simulink model "Research_project_CSTR_cascade"  (R2022b)
settings: Solver=ode23s  StartTime=0.0  StopTime=360  RelTol=1e-3
model workspace (MAT data in the model file):
  Var = 0
undefined symbols (not defined in the file): A, CA0, FA0, Tfeed, Tfeedout, Tj, U, V, v0, Xin, Xout
(part 2 of 2)

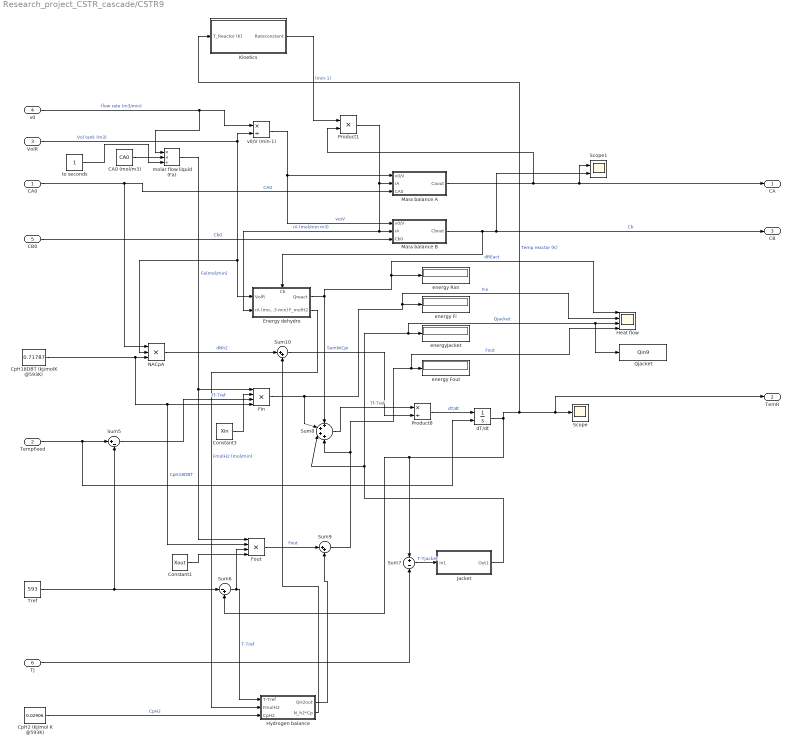
== system Research_project_CSTR_cascade/CSTR9 ==
  CA0 : Inport
  TempFeed : Inport  Port=2
  VolR : Inport  Port=3
  v0 : Inport  Port=4
  CB0 : Inport  Port=5
  Tj : Inport  Port=6
  CA0 (mol/m3) : Constant  Value=CA0
  Constant1 : Constant  Value=Xout
  Constant3 : Constant  Value=Xin
  CpH18DBT (kj/molK @593K) : Constant  Value=0.71787
  CpH2 (kj/mol K @593K) : Constant  Value=0.02906
  Energy dehydro : Subsystem
      settings: PortSchema="{\"entries\":[{\"content\":{\"sides\":[{\"content\":{\"connectorIds\":[\"In1\",\"In2\"]},\"type\":\"ConnectorPlacement.EquallySpacedRectSide\",\"uuid\":\"ea2ca829-97b9-403b-8ba1-0454ae3e30fe\"},{\"content\":{\"connectorIds\":[\"Out1\",\"Out2\"],\"side\":\"RIGHT\"},\"type\":\"ConnectorPlacement.EquallySpacedRectSide\",\"uuid\":\"58c9b242-3f0e-4d7f-8153-41ceacc042f7\"},{\"content\":{\"connectorIds\":[\"In3\"],\"side\":\"TOP\"},\"type\":\"ConnectorPlacement.EquallySpacedRectSide\",\"uuid\":\"130a98c9-d360-4861-8a60-9ab6de0c7020\"}]},\"type\":\"ConnectorPlacement.EquallySpacedConnector\",\"uuid\":\"a36fbf0c-f6b7-4cf9-83b8-7faebe270894\"}],\"packageUris\":[\"http://schema.mathworks.com/mf0/Connector/R2020b\"],\"version\":\"1.0\"}"
  Fin : Product  Inputs=4
  Fout : Product  Inputs=4
  Heat flow : Scope  NumInputPorts=4
  Hydrogen balance : Subsystem
  Jacket : Subsystem
  Kinetics : Subsystem
  Mass balance A : Subsystem
  Mass balance B : Subsystem
  NACpA : Product  Inputs=3
  Product1 : Product
  Product8 : Product  Inputs=*/
  Qjacket : ToWorkspace  VariableName=Qin9  SaveFormat=Timeseries  SampleTime=1
  Scope : Scope
  Scope1 : Scope  NumInputPorts=2
  Sum10 : Sum  Inputs=|++
  Sum5 : Sum  Inputs=|+-
  Sum6 : Sum  Inputs=|-+
  Sum7 : Sum  Inputs=+-
  Sum8 : Sum  Inputs=++++
  Sum9 : Sum  Inputs=|++
  Tref : Constant  Value=593
  dT/dt : Integrator  InitialConditionSource=external  InitialCondition=593
  energy Fi : Display
  energy Fout : Display
  energy Rxn : Display
  energyJacket : Display
  molar flow liquid (Fa) : Product  Inputs=**/
  to seconds : Constant
  v0/V (min-1) : Product  Inputs=*/
  CA : Outport
  TemR : Outport  Port=2
  CB : Outport  Port=3
  wires:
  VolR/1 -> Energy dehydro/1(VolR), NACpA/2, v0/V (min-1)/2  "Vol tank (m3)"
  v0/1 -> v0/V (min-1)/1, molar flow liquid (Fa)/1  "flow rate (m3/min)"
  CA0/1 -> NACpA/1, Mass balance A/3(CA0)  "CA0"
  Product1/1 -> Mass balance A/2(rA), Energy dehydro/2(rA (mol/m3 min)), Mass balance B/2(rA)  "rA (mol/min m3)"
  CB0/1 -> Mass balance B/3(Cb0)  "Cb0"
  v0/V (min-1)/1 -> Mass balance B/1(v0/V), Mass balance A/1(v0/V)  "vo/V"
  Mass balance B/1(Cbout) -> CB/1, Scope1/2, Energy dehydro/3(Cb)  "Cb"
  CpH18DBT (kj/molK @593K)/1 -> NACpA/3, Fin/4, Fout/2  "CpH18DBT"
  Tref/1 -> Sum5/2, Sum6/1
  Sum5/1 -> Fin/3  "Tf-Tref"
  to seconds/1 -> molar flow liquid (Fa)/3
  molar flow liquid (Fa)/1 -> Fout/1, Fin/1  "Fa(mol/min)"
  dT/dt/1 -> Kinetics/1(T_Reactor (K)), TemR/1, Scope/1, Sum6/2, Sum7/1  "Temp reactor (K)"
  Sum6/1 -> Hydrogen balance/1(T-Tref), Fout/3  "T-Tref"
  Tj/1 -> Sum7/2
  Jacket/1(Out1) -> Qjacket/1, Heat flow/3, energyJacket/1, Sum8/3  "Qjacket"
  Fin/1 -> Heat flow/2, energy Fi/1, Sum8/2  "Fin"
  Sum9/1 -> Heat flow/4, energy Fout/1, Sum8/4  "Fout"
  Energy dehydro/1(Qreact) -> Sum8/1, Heat flow/1, energy Rxn/1  "dREact"
  Sum8/1 -> Product8/1  "Tf-Tref"
  Product8/1 -> dT/dt/1  "dT/dt"
  Constant1/1 -> Fout/4
  TempFeed/1 -> dT/dt/2, Sum5/1
  Kinetics/1(Rateconstant) -> Product1/1  "(min-1)"
  Constant3/1 -> Fin/2
  CpH2 (kj/mol K @593K)/1 -> Hydrogen balance/3(CpH2)  "CpH2"
  Energy dehydro/2(F_molH2) -> Hydrogen balance/2(FmolH2)  "FmolH2 (mol/min)"
  Fout/1 -> Sum9/1  "Fout"
  Sum7/1 -> Jacket/1(In1)  "T-Tjacket"
  Hydrogen balance/1(QH2out) -> Sum9/2
  NACpA/1 -> Sum10/1  "dNh2"
  Sum10/1 -> Product8/2  "SumNiCpi"
  Hydrogen balance/2(N_h2*Cp) -> Sum10/2
  Mass balance A/1(Caout) -> Scope1/1, CA/1, Product1/2
  CA0 (mol/m3)/1 -> molar flow liquid (Fa)/2

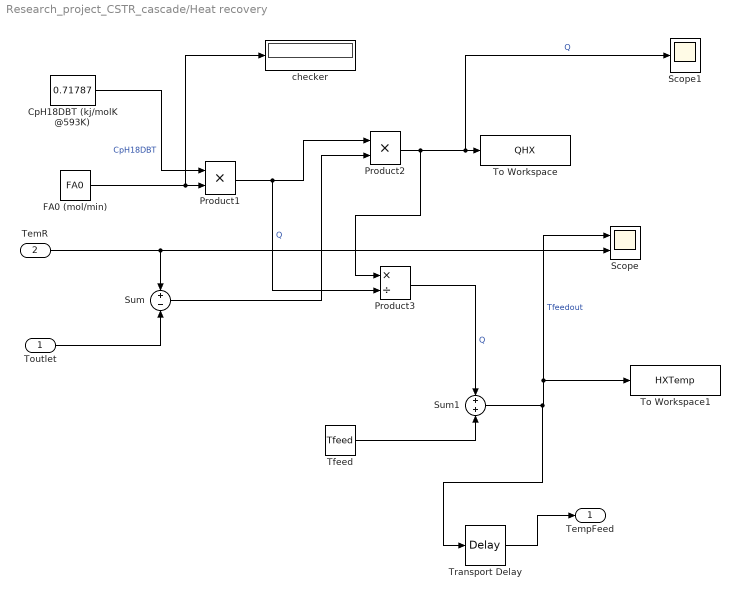
== system Research_project_CSTR_cascade/Heat recovery ==
  Toutlet : Inport
  TemR : Inport  Port=2
  CpH18DBT (kj/molK @593K) : Constant  Value=0.71787
  FA0 (mol/min) : Constant  Value=FA0
  Product1 : Product
  Product2 : Product
  Product3 : Product  Inputs=*/
  Scope : Scope  NumInputPorts=2
  Scope1 : Scope
  Sum : Sum  Inputs=+-
  Sum1 : Sum
  Tfeed : Constant  Value=Tfeed
  To Workspace : ToWorkspace  VariableName=QHX  SaveFormat=Timeseries  SampleTime=1
  To Workspace1 : ToWorkspace  VariableName=HXTemp  SaveFormat=Timeseries  SampleTime=5
  Transport Delay : TransportDelay
  checker : Display
  TempFeed : Outport
  wires:
  TemR/1 -> Sum/1, Scope/2
  FA0 (mol/min)/1 -> checker/1, Product1/2
  Sum/1 -> Product2/2
  CpH18DBT (kj/molK @593K)/1 -> Product1/1  "CpH18DBT"
  Product2/1 -> Product3/1, Scope1/1, To Workspace/1  "Q"
  Product1/1 -> Product3/2, Product2/1  "Q"
  Tfeed/1 -> Sum1/2
  Product3/1 -> Sum1/1  "Q"
  Sum1/1 -> Transport Delay/1, To Workspace1/1, Scope/1  "Tfeedout"
  Transport Delay/1 -> TempFeed/1
  Toutlet/1 -> Sum/2

== system Research_project_CSTR_cascade/mol ==
  V : Inport
  Cb : Inport  Port=2
  CA : Inport  Port=3
  Constant : Constant  Value=9
  Product : Product
  Product1 : Product
  Product2 : Product
  H2 : Outport
  H0DBT : Outport  Port=2
  H18DBT : Outport  Port=3
  wires:
  Product1/1 -> H0DBT/1, Product2/2  "H0DBT"
  Constant/1 -> Product2/1
  Product/1 -> H18DBT/1  "H18DBT"
  Product2/1 -> H2/1  "H2"
  V/1 -> Product1/1, Product/1  "V"
  CA/1 -> Product/2  "Conc H18-DBT"
  Cb/1 -> Product1/2

== system Research_project_CSTR_cascade/CSTR1/Energy dehydro ==
  VolR : Inport
  rA (mol/m3 min) : Inport  Port=2
  Cb : Inport  Port=3
  9H2 : Constant  Value=9
  Product1 : Product  Inputs=3
  Product2 : Product  Inputs=3
  Product6 : Product
  reaction enth (kj/molH2) : Constant  Value=-64
  Qreact : Outport
  F_molH2 : Outport  Port=2
  wires:
  9H2/1 -> Product2/2, Product1/3
  VolR/1 -> Product2/1, Product1/1
  rA (mol/m3 min)/1 -> Product1/2
  reaction enth (kj/molH2)/1 -> Product6/2
  Product1/1 -> F_molH2/1, Product6/1  "rA rate of H2 react (mol of H2/min)"
  Product6/1 -> Qreact/1  "dREact"
  Cb/1 -> Product2/3  "mol/m3min"

== system Research_project_CSTR_cascade/CSTR1/Hydrogen balance ==
  T-Tref : Inport
  FmolH2 : Inport  Port=2
  CpH2 : Inport  Port=3
  Constant1 : Constant  Value=Xout
  FoutH2CpdT2 : Product  Inputs=4
  N_H2*Cp : Product
  Scope1 : Scope
  QH2out : Outport
  N_h2*Cp : Outport  Port=2
  wires:
  FoutH2CpdT2/1 -> Scope1/1, QH2out/1  "QH2"
  T-Tref/1 -> FoutH2CpdT2/1
  CpH2/1 -> N_H2*Cp/2, FoutH2CpdT2/2
  FmolH2/1 -> N_H2*Cp/1, FoutH2CpdT2/3
  N_H2*Cp/1 -> N_h2*Cp/1  "QH2"
  Constant1/1 -> FoutH2CpdT2/4

== system Research_project_CSTR_cascade/CSTR1/Jacket ==
  In1 : Inport
  Area Heat (m2) : Constant  Value=A
  Q : Product  Inputs=3
  U (Kj/min m2 K) : Constant  Value=U
  Out1 : Outport
  wires:
  Area Heat (m2)/1 -> Q/3  "A jacket (m2)"
  U (Kj/min m2 K)/1 -> Q/1
  In1/1 -> Q/2  "T-Tjacket"
  Q/1 -> Out1/1  "Qjacket"

== system Research_project_CSTR_cascade/CSTR1/Kinetics ==
  T_Reactor (K) : Inport
  "A constant " : Math
  Constant : Constant  Value=37.634
  Ea (kj/mol) : Constant  Value=-204.68
  Effectiveness factor : Constant
  Math Function : Math
  Product3 : Product
  Product4 : Product  Inputs=3
  Product5 : Product  Inputs=*/
  R (kj/mol K) : Constant  Value=0.00831
  Rateconstant : Outport
  wires:
  T_Reactor (K)/1 -> Product3/1
  "A constant "/1 -> Product4/1
  Product3/1 -> Product5/2
  Constant/1 -> "A constant "/1
  Ea (kj/mol)/1 -> Product5/1
  Math Function/1 -> Product4/2
  R (kj/mol K)/1 -> Product3/2
  Product5/1 -> Math Function/1
  Product4/1 -> Rateconstant/1  "(min-1)"
  Effectiveness factor/1 -> Product4/3

== system Research_project_CSTR_cascade/CSTR1/Mass balance A ==
  v0/V : Inport
  rA : Inport  Port=2
  CA0 : Inport  Port=3
  Product1 : Product
  Scope : Scope
  Sum1 : Sum  Inputs=|+-
  Sum2 : Sum  Inputs=|+-
  dCa/dt : Integrator  InitialConditionSource=external  InitialCondition=3100
  Caout : Outport
  wires:
  rA/1 -> Sum2/2  "rA (mol/min m3)"
  Sum2/1 -> dCa/dt/1
  CA0/1 -> dCa/dt/2, Sum1/1
  Product1/1 -> Sum2/1
  dCa/dt/1 -> Scope/1, Caout/1, Sum1/2  "Ca (mol/m3 min)"
  Sum1/1 -> Product1/2  "Ca0-Ca"
  v0/V/1 -> Product1/1

== system Research_project_CSTR_cascade/CSTR1/Mass balance B ==
  v0/V : Inport
  rA : Inport  Port=2
  Cb0 : Inport  Port=3
  Product1 : Product
  Scope : Scope
  Sum1 : Sum  Inputs=|+-
  Sum2 : Sum  Inputs=|++
  dCb/dt : Integrator  InitialConditionSource=external  InitialCondition=3100
  Cbout : Outport
  wires:
  rA/1 -> Sum2/2  "rA (mol/min m3)"
  Sum2/1 -> dCb/dt/1
  Cb0/1 -> dCb/dt/2, Sum1/1
  Product1/1 -> Sum2/1
  dCb/dt/1 -> Scope/1, Cbout/1, Sum1/2  "Cb (mol/m3 min)"
  Sum1/1 -> Product1/2  "Cb0-Cb"
  v0/V/1 -> Product1/1

== system Research_project_CSTR_cascade/CSTR10/Energy dehydro ==
  VolR : Inport
  rA (mol/m3 min) : Inport  Port=2
  9H2 : Constant  Value=9
  B : Constant
  Product1 : Product  Inputs=3
  Product2 : Product  Inputs=3
  Product6 : Product
  Qjacket : ToWorkspace  VariableName=H2  SaveFormat=Timeseries  SampleTime=5
  Scope1 : Scope  NumInputPorts=2
  reaction enth (kj/molH2) : Constant  Value=-64
  Qreact : Outport
  F_molH2 : Outport  Port=2
  wires:
  9H2/1 -> Product1/3
  VolR/1 -> Product2/1, Product1/1
  rA (mol/m3 min)/1 -> Product2/2, Product1/2
  reaction enth (kj/molH2)/1 -> Product6/2
  Product6/1 -> Qreact/1  "dREact"
  Product1/1 -> Qjacket/1, Scope1/2, F_molH2/1, Product6/1  "mol of H2"
  Product2/1 -> Scope1/1  "mol H0-DBT"
  B/1 -> Product2/3

== system Research_project_CSTR_cascade/CSTR10/Hydrogen balance ==
  T-Tref : Inport
  FmolH2 : Inport  Port=2
  CpH2 : Inport  Port=3
  Constant1 : Constant  Value=Xout
  FoutH2CpdT2 : Product  Inputs=4
  N_H2*Cp : Product
  Scope1 : Scope
  QH2out : Outport
  N_h2*Cp : Outport  Port=2
  wires:
  FoutH2CpdT2/1 -> Scope1/1, QH2out/1  "QH2"
  T-Tref/1 -> FoutH2CpdT2/1
  CpH2/1 -> N_H2*Cp/2, FoutH2CpdT2/2
  FmolH2/1 -> N_H2*Cp/1, FoutH2CpdT2/3
  N_H2*Cp/1 -> N_h2*Cp/1  "QH2"
  Constant1/1 -> FoutH2CpdT2/4

== system Research_project_CSTR_cascade/CSTR10/Jacket ==
  In1 : Inport
  Area Heat (m2) : Constant  Value=A
  Q : Product  Inputs=3
  U (Kj/min m2 K) : Constant  Value=U
  Out1 : Outport
  wires:
  Area Heat (m2)/1 -> Q/3  "A jacket (m2)"
  U (Kj/min m2 K)/1 -> Q/1
  In1/1 -> Q/2  "T-Tjacket"
  Q/1 -> Out1/1  "Qjacket"

== system Research_project_CSTR_cascade/CSTR10/Kinetics ==
  T_Reactor (K) : Inport
  "A constant " : Math
  Constant : Constant  Value=37.634
  Ea (kj/mol) : Constant  Value=-204.68
  Effectiveness factor : Constant
  Math Function : Math
  Product3 : Product
  Product4 : Product  Inputs=3
  Product5 : Product  Inputs=*/
  R (kj/mol K) : Constant  Value=0.00831
  Rateconstant : Outport
  wires:
  T_Reactor (K)/1 -> Product3/1
  "A constant "/1 -> Product4/1
  Product3/1 -> Product5/2
  Constant/1 -> "A constant "/1
  Ea (kj/mol)/1 -> Product5/1
  Math Function/1 -> Product4/2
  R (kj/mol K)/1 -> Product3/2
  Product5/1 -> Math Function/1
  Product4/1 -> Rateconstant/1  "(min-1)"
  Effectiveness factor/1 -> Product4/3

== system Research_project_CSTR_cascade/CSTR10/Mass balance A ==
  v0/V : Inport
  rA : Inport  Port=2
  CA0 : Inport  Port=3
  Product1 : Product
  Scope : Scope
  Sum1 : Sum  Inputs=|+-
  Sum2 : Sum  Inputs=|+-
  dCa/dt : Integrator  InitialConditionSource=external  InitialCondition=3100
  Caout : Outport
  wires:
  rA/1 -> Sum2/2  "rA (mol/min m3)"
  Sum2/1 -> dCa/dt/1
  CA0/1 -> dCa/dt/2, Sum1/1
  Product1/1 -> Sum2/1
  dCa/dt/1 -> Scope/1, Caout/1, Sum1/2  "Ca (mol/m3 min)"
  Sum1/1 -> Product1/2  "Ca0-Ca"
  v0/V/1 -> Product1/1

== system Research_project_CSTR_cascade/CSTR10/Mass balance B ==
  v0/V : Inport
  rA : Inport  Port=2
  Cb0 : Inport  Port=3
  Product1 : Product
  Scope : Scope
  Sum1 : Sum  Inputs=|+-
  Sum2 : Sum  Inputs=|++
  dCb/dt : Integrator  InitialConditionSource=external  InitialCondition=3100
  Cbout : Outport
  wires:
  rA/1 -> Sum2/2  "rA (mol/min m3)"
  Sum2/1 -> dCb/dt/1
  Cb0/1 -> dCb/dt/2, Sum1/1
  Product1/1 -> Sum2/1
  dCb/dt/1 -> Scope/1, Cbout/1, Sum1/2  "Cb (mol/m3 min)"
  Sum1/1 -> Product1/2  "Cb0-Cb"
  v0/V/1 -> Product1/1

== system Research_project_CSTR_cascade/CSTR2/Energy dehydro ==
  VolR : Inport
  rA (mol/m3 min) : Inport  Port=2
  Cb : Inport  Port=3
  9H2 : Constant  Value=9
  Product1 : Product  Inputs=3
  Product2 : Product  Inputs=3
  Product6 : Product
  reaction enth (kj/molH2) : Constant  Value=-64
  Qreact : Outport
  F_molH2 : Outport  Port=2
  wires:
  9H2/1 -> Product2/2, Product1/3
  VolR/1 -> Product2/1, Product1/1
  rA (mol/m3 min)/1 -> Product1/2
  reaction enth (kj/molH2)/1 -> Product6/2
  Product1/1 -> F_molH2/1, Product6/1  "rA rate of H2 react (mol of H2/min)"
  Product6/1 -> Qreact/1  "dREact"
  Cb/1 -> Product2/3  "mol/m3min"

== system Research_project_CSTR_cascade/CSTR2/Hydrogen balance ==
  T-Tref : Inport
  FmolH2 : Inport  Port=2
  CpH2 : Inport  Port=3
  Constant1 : Constant  Value=Xout
  FoutH2CpdT2 : Product  Inputs=4
  N_H2*Cp : Product
  Scope1 : Scope
  QH2out : Outport
  N_h2*Cp : Outport  Port=2
  wires:
  FoutH2CpdT2/1 -> Scope1/1, QH2out/1  "QH2"
  T-Tref/1 -> FoutH2CpdT2/1
  CpH2/1 -> N_H2*Cp/2, FoutH2CpdT2/2
  FmolH2/1 -> N_H2*Cp/1, FoutH2CpdT2/3
  N_H2*Cp/1 -> N_h2*Cp/1  "QH2"
  Constant1/1 -> FoutH2CpdT2/4

== system Research_project_CSTR_cascade/CSTR2/Jacket ==
  In1 : Inport
  Area Heat (m2) : Constant  Value=A
  Q : Product  Inputs=3
  U (Kj/min m2 K) : Constant  Value=U
  Out1 : Outport
  wires:
  Area Heat (m2)/1 -> Q/3  "A jacket (m2)"
  U (Kj/min m2 K)/1 -> Q/1
  In1/1 -> Q/2  "T-Tjacket"
  Q/1 -> Out1/1  "Qjacket"

== system Research_project_CSTR_cascade/CSTR2/Kinetics ==
  T_Reactor (K) : Inport
  "A constant " : Math
  Constant : Constant  Value=37.634
  Ea (kj/mol) : Constant  Value=-204.68
  Effectiveness factor : Constant
  Math Function : Math
  Product3 : Product
  Product4 : Product  Inputs=3
  Product5 : Product  Inputs=*/
  R (kj/mol K) : Constant  Value=0.00831
  Rateconstant : Outport
  wires:
  T_Reactor (K)/1 -> Product3/1
  "A constant "/1 -> Product4/1
  Product3/1 -> Product5/2
  Constant/1 -> "A constant "/1
  Ea (kj/mol)/1 -> Product5/1
  Math Function/1 -> Product4/2
  R (kj/mol K)/1 -> Product3/2
  Product5/1 -> Math Function/1
  Product4/1 -> Rateconstant/1  "(min-1)"
  Effectiveness factor/1 -> Product4/3

== system Research_project_CSTR_cascade/CSTR2/Mass balance A ==
  v0/V : Inport
  rA : Inport  Port=2
  CA0 : Inport  Port=3
  Product1 : Product
  Scope : Scope
  Sum1 : Sum  Inputs=|+-
  Sum2 : Sum  Inputs=|+-
  dCa/dt : Integrator  InitialConditionSource=external  InitialCondition=3100
  Caout : Outport
  wires:
  rA/1 -> Sum2/2  "rA (mol/min m3)"
  Sum2/1 -> dCa/dt/1
  CA0/1 -> dCa/dt/2, Sum1/1
  Product1/1 -> Sum2/1
  dCa/dt/1 -> Scope/1, Caout/1, Sum1/2  "Ca (mol/m3 min)"
  Sum1/1 -> Product1/2  "Ca0-Ca"
  v0/V/1 -> Product1/1

== system Research_project_CSTR_cascade/CSTR2/Mass balance B ==
  v0/V : Inport
  rA : Inport  Port=2
  Cb0 : Inport  Port=3
  Product1 : Product
  Scope : Scope
  Sum1 : Sum  Inputs=|+-
  Sum2 : Sum  Inputs=|++
  dCb/dt : Integrator  InitialConditionSource=external  InitialCondition=3100
  Cbout : Outport
  wires:
  rA/1 -> Sum2/2  "rA (mol/min m3)"
  Sum2/1 -> dCb/dt/1
  Cb0/1 -> dCb/dt/2, Sum1/1
  Product1/1 -> Sum2/1
  dCb/dt/1 -> Scope/1, Cbout/1, Sum1/2  "Cb (mol/m3 min)"
  Sum1/1 -> Product1/2  "Cb0-Cb"
  v0/V/1 -> Product1/1

== system Research_project_CSTR_cascade/CSTR3/Energy dehydro ==
  VolR : Inport
  rA (mol/m3 min) : Inport  Port=2
  Cb : Inport  Port=3
  9H2 : Constant  Value=9
  Product1 : Product  Inputs=3
  Product2 : Product  Inputs=3
  Product6 : Product
  reaction enth (kj/molH2) : Constant  Value=-64
  Qreact : Outport
  F_molH2 : Outport  Port=2
  wires:
  9H2/1 -> Product2/2, Product1/3
  VolR/1 -> Product2/1, Product1/1
  rA (mol/m3 min)/1 -> Product1/2
  reaction enth (kj/molH2)/1 -> Product6/2
  Product1/1 -> F_molH2/1, Product6/1  "rA rate of H2 react (mol of H2/min)"
  Product6/1 -> Qreact/1  "dREact"
  Cb/1 -> Product2/3  "mol/m3min"

== system Research_project_CSTR_cascade/CSTR3/Hydrogen balance ==
  T-Tref : Inport
  FmolH2 : Inport  Port=2
  CpH2 : Inport  Port=3
  Constant1 : Constant  Value=Xout
  FoutH2CpdT2 : Product  Inputs=4
  N_H2*Cp : Product
  Scope1 : Scope
  QH2out : Outport
  N_h2*Cp : Outport  Port=2
  wires:
  FoutH2CpdT2/1 -> Scope1/1, QH2out/1  "QH2"
  T-Tref/1 -> FoutH2CpdT2/1
  CpH2/1 -> N_H2*Cp/2, FoutH2CpdT2/2
  FmolH2/1 -> N_H2*Cp/1, FoutH2CpdT2/3
  N_H2*Cp/1 -> N_h2*Cp/1  "QH2"
  Constant1/1 -> FoutH2CpdT2/4

== system Research_project_CSTR_cascade/CSTR3/Jacket ==
  In1 : Inport
  Area Heat (m2) : Constant  Value=A
  Q : Product  Inputs=3
  U (Kj/min m2 K) : Constant  Value=U
  Out1 : Outport
  wires:
  Area Heat (m2)/1 -> Q/3  "A jacket (m2)"
  U (Kj/min m2 K)/1 -> Q/1
  In1/1 -> Q/2  "T-Tjacket"
  Q/1 -> Out1/1  "Qjacket"

== system Research_project_CSTR_cascade/CSTR3/Kinetics ==
  T_Reactor (K) : Inport
  "A constant " : Math
  Constant : Constant  Value=37.634
  Ea (kj/mol) : Constant  Value=-204.68
  Effectiveness factor : Constant
  Math Function : Math
  Product3 : Product
  Product4 : Product  Inputs=3
  Product5 : Product  Inputs=*/
  R (kj/mol K) : Constant  Value=0.00831
  Rateconstant : Outport
  wires:
  T_Reactor (K)/1 -> Product3/1
  "A constant "/1 -> Product4/1
  Product3/1 -> Product5/2
  Constant/1 -> "A constant "/1
  Ea (kj/mol)/1 -> Product5/1
  Math Function/1 -> Product4/2
  R (kj/mol K)/1 -> Product3/2
  Product5/1 -> Math Function/1
  Product4/1 -> Rateconstant/1  "(min-1)"
  Effectiveness factor/1 -> Product4/3

== system Research_project_CSTR_cascade/CSTR3/Mass balance A ==
  v0/V : Inport
  rA : Inport  Port=2
  CA0 : Inport  Port=3
  Product1 : Product
  Scope : Scope
  Sum1 : Sum  Inputs=|+-
  Sum2 : Sum  Inputs=|+-
  dCa/dt : Integrator  InitialConditionSource=external  InitialCondition=3100
  Caout : Outport
  wires:
  rA/1 -> Sum2/2  "rA (mol/min m3)"
  Sum2/1 -> dCa/dt/1
  CA0/1 -> dCa/dt/2, Sum1/1
  Product1/1 -> Sum2/1
  dCa/dt/1 -> Scope/1, Caout/1, Sum1/2  "Ca (mol/m3 min)"
  Sum1/1 -> Product1/2  "Ca0-Ca"
  v0/V/1 -> Product1/1

== system Research_project_CSTR_cascade/CSTR3/Mass balance B ==
  v0/V : Inport
  rA : Inport  Port=2
  Cb0 : Inport  Port=3
  Product1 : Product
  Scope : Scope
  Sum1 : Sum  Inputs=|+-
  Sum2 : Sum  Inputs=|++
  dCb/dt : Integrator  InitialConditionSource=external  InitialCondition=3100
  Cbout : Outport
  wires:
  rA/1 -> Sum2/2  "rA (mol/min m3)"
  Sum2/1 -> dCb/dt/1
  Cb0/1 -> dCb/dt/2, Sum1/1
  Product1/1 -> Sum2/1
  dCb/dt/1 -> Scope/1, Cbout/1, Sum1/2  "Cb (mol/m3 min)"
  Sum1/1 -> Product1/2  "Cb0-Cb"
  v0/V/1 -> Product1/1

== system Research_project_CSTR_cascade/CSTR4/Energy dehydro ==
  VolR : Inport
  rA (mol/m3 min) : Inport  Port=2
  Cb : Inport  Port=3
  9H2 : Constant  Value=9
  Product1 : Product  Inputs=3
  Product2 : Product  Inputs=3
  Product6 : Product
  reaction enth (kj/molH2) : Constant  Value=-64
  Qreact : Outport
  F_molH2 : Outport  Port=2
  wires:
  9H2/1 -> Product2/2, Product1/3
  VolR/1 -> Product2/1, Product1/1
  rA (mol/m3 min)/1 -> Product1/2
  reaction enth (kj/molH2)/1 -> Product6/2
  Product1/1 -> F_molH2/1, Product6/1  "rA rate of H2 react (mol of H2/min)"
  Product6/1 -> Qreact/1  "dREact"
  Cb/1 -> Product2/3  "mol/m3min"

== system Research_project_CSTR_cascade/CSTR4/Hydrogen balance ==
  T-Tref : Inport
  FmolH2 : Inport  Port=2
  CpH2 : Inport  Port=3
  Constant1 : Constant  Value=Xout
  FoutH2CpdT2 : Product  Inputs=4
  N_H2*Cp : Product
  Scope1 : Scope
  QH2out : Outport
  N_h2*Cp : Outport  Port=2
  wires:
  FoutH2CpdT2/1 -> Scope1/1, QH2out/1  "QH2"
  T-Tref/1 -> FoutH2CpdT2/1
  CpH2/1 -> N_H2*Cp/2, FoutH2CpdT2/2
  FmolH2/1 -> N_H2*Cp/1, FoutH2CpdT2/3
  N_H2*Cp/1 -> N_h2*Cp/1  "QH2"
  Constant1/1 -> FoutH2CpdT2/4

== system Research_project_CSTR_cascade/CSTR4/Jacket ==
  In1 : Inport
  Area Heat (m2) : Constant  Value=A
  Q : Product  Inputs=3
  U (Kj/min m2 K) : Constant  Value=U
  Out1 : Outport
  wires:
  Area Heat (m2)/1 -> Q/3  "A jacket (m2)"
  U (Kj/min m2 K)/1 -> Q/1
  In1/1 -> Q/2  "T-Tjacket"
  Q/1 -> Out1/1  "Qjacket"

== system Research_project_CSTR_cascade/CSTR4/Kinetics ==
  T_Reactor (K) : Inport
  "A constant " : Math
  Constant : Constant  Value=37.634
  Ea (kj/mol) : Constant  Value=-204.68
  Effectiveness factor : Constant
  Math Function : Math
  Product3 : Product
  Product4 : Product  Inputs=3
  Product5 : Product  Inputs=*/
  R (kj/mol K) : Constant  Value=0.00831
  Rateconstant : Outport
  wires:
  T_Reactor (K)/1 -> Product3/1
  "A constant "/1 -> Product4/1
  Product3/1 -> Product5/2
  Constant/1 -> "A constant "/1
  Ea (kj/mol)/1 -> Product5/1
  Math Function/1 -> Product4/2
  R (kj/mol K)/1 -> Product3/2
  Product5/1 -> Math Function/1
  Product4/1 -> Rateconstant/1  "(min-1)"
  Effectiveness factor/1 -> Product4/3

== system Research_project_CSTR_cascade/CSTR4/Mass balance A ==
  v0/V : Inport
  rA : Inport  Port=2
  CA0 : Inport  Port=3
  Product1 : Product
  Scope : Scope
  Sum1 : Sum  Inputs=|+-
  Sum2 : Sum  Inputs=|+-
  dCa/dt : Integrator  InitialConditionSource=external  InitialCondition=3100
  Caout : Outport
  wires:
  rA/1 -> Sum2/2  "rA (mol/min m3)"
  Sum2/1 -> dCa/dt/1
  CA0/1 -> dCa/dt/2, Sum1/1
  Product1/1 -> Sum2/1
  dCa/dt/1 -> Scope/1, Caout/1, Sum1/2  "Ca (mol/m3 min)"
  Sum1/1 -> Product1/2  "Ca0-Ca"
  v0/V/1 -> Product1/1

== system Research_project_CSTR_cascade/CSTR4/Mass balance B ==
  v0/V : Inport
  rA : Inport  Port=2
  Cb0 : Inport  Port=3
  Product1 : Product
  Scope : Scope
  Sum1 : Sum  Inputs=|+-
  Sum2 : Sum  Inputs=|++
  dCb/dt : Integrator  InitialConditionSource=external  InitialCondition=3100
  Cbout : Outport
  wires:
  rA/1 -> Sum2/2  "rA (mol/min m3)"
  Sum2/1 -> dCb/dt/1
  Cb0/1 -> dCb/dt/2, Sum1/1
  Product1/1 -> Sum2/1
  dCb/dt/1 -> Scope/1, Cbout/1, Sum1/2  "Cb (mol/m3 min)"
  Sum1/1 -> Product1/2  "Cb0-Cb"
  v0/V/1 -> Product1/1

== system Research_project_CSTR_cascade/CSTR5/Energy dehydro ==
  VolR : Inport
  rA (mol/m3 min) : Inport  Port=2
  Cb : Inport  Port=3
  9H2 : Constant  Value=9
  Product1 : Product  Inputs=3
  Product2 : Product  Inputs=3
  Product6 : Product
  reaction enth (kj/molH2) : Constant  Value=-64
  Qreact : Outport
  F_molH2 : Outport  Port=2
  wires:
  9H2/1 -> Product2/2, Product1/3
  VolR/1 -> Product2/1, Product1/1
  rA (mol/m3 min)/1 -> Product1/2
  reaction enth (kj/molH2)/1 -> Product6/2
  Product1/1 -> F_molH2/1, Product6/1  "rA rate of H2 react (mol of H2/min)"
  Product6/1 -> Qreact/1  "dREact"
  Cb/1 -> Product2/3  "mol/m3min"

== system Research_project_CSTR_cascade/CSTR5/Hydrogen balance ==
  T-Tref : Inport
  FmolH2 : Inport  Port=2
  CpH2 : Inport  Port=3
  Constant1 : Constant  Value=Xout
  FoutH2CpdT2 : Product  Inputs=4
  N_H2*Cp : Product
  Scope1 : Scope
  QH2out : Outport
  N_h2*Cp : Outport  Port=2
  wires:
  FoutH2CpdT2/1 -> Scope1/1, QH2out/1  "QH2"
  T-Tref/1 -> FoutH2CpdT2/1
  CpH2/1 -> N_H2*Cp/2, FoutH2CpdT2/2
  FmolH2/1 -> N_H2*Cp/1, FoutH2CpdT2/3
  N_H2*Cp/1 -> N_h2*Cp/1  "QH2"
  Constant1/1 -> FoutH2CpdT2/4

== system Research_project_CSTR_cascade/CSTR5/Jacket ==
  In1 : Inport
  Area Heat (m2) : Constant  Value=A
  Q : Product  Inputs=3
  U (Kj/min m2 K) : Constant  Value=U
  Out1 : Outport
  wires:
  Area Heat (m2)/1 -> Q/3  "A jacket (m2)"
  U (Kj/min m2 K)/1 -> Q/1
  In1/1 -> Q/2  "T-Tjacket"
  Q/1 -> Out1/1  "Qjacket"

== system Research_project_CSTR_cascade/CSTR5/Kinetics ==
  T_Reactor (K) : Inport
  "A constant " : Math
  Constant : Constant  Value=37.634
  Ea (kj/mol) : Constant  Value=-204.68
  Effectiveness factor : Constant
  Math Function : Math
  Product3 : Product
  Product4 : Product  Inputs=3
  Product5 : Product  Inputs=*/
  R (kj/mol K) : Constant  Value=0.00831
  Rateconstant : Outport
  wires:
  T_Reactor (K)/1 -> Product3/1
  "A constant "/1 -> Product4/1
  Product3/1 -> Product5/2
  Constant/1 -> "A constant "/1
  Ea (kj/mol)/1 -> Product5/1
  Math Function/1 -> Product4/2
  R (kj/mol K)/1 -> Product3/2
  Product5/1 -> Math Function/1
  Product4/1 -> Rateconstant/1  "(min-1)"
  Effectiveness factor/1 -> Product4/3

== system Research_project_CSTR_cascade/CSTR5/Mass balance A ==
  v0/V : Inport
  rA : Inport  Port=2
  CA0 : Inport  Port=3
  Product1 : Product
  Scope : Scope
  Sum1 : Sum  Inputs=|+-
  Sum2 : Sum  Inputs=|+-
  dCa/dt : Integrator  InitialConditionSource=external  InitialCondition=3100
  Caout : Outport
  wires:
  rA/1 -> Sum2/2  "rA (mol/min m3)"
  Sum2/1 -> dCa/dt/1
  CA0/1 -> dCa/dt/2, Sum1/1
  Product1/1 -> Sum2/1
  dCa/dt/1 -> Scope/1, Caout/1, Sum1/2  "Ca (mol/m3 min)"
  Sum1/1 -> Product1/2  "Ca0-Ca"
  v0/V/1 -> Product1/1

== system Research_project_CSTR_cascade/CSTR5/Mass balance B ==
  v0/V : Inport
  rA : Inport  Port=2
  Cb0 : Inport  Port=3
  Product1 : Product
  Scope : Scope
  Sum1 : Sum  Inputs=|+-
  Sum2 : Sum  Inputs=|++
  dCb/dt : Integrator  InitialConditionSource=external  InitialCondition=3100
  Cbout : Outport
  wires:
  rA/1 -> Sum2/2  "rA (mol/min m3)"
  Sum2/1 -> dCb/dt/1
  Cb0/1 -> dCb/dt/2, Sum1/1
  Product1/1 -> Sum2/1
  dCb/dt/1 -> Scope/1, Cbout/1, Sum1/2  "Cb (mol/m3 min)"
  Sum1/1 -> Product1/2  "Cb0-Cb"
  v0/V/1 -> Product1/1

== system Research_project_CSTR_cascade/CSTR6/Energy dehydro ==
  VolR : Inport
  rA (mol/m3 min) : Inport  Port=2
  Cb : Inport  Port=3
  9H2 : Constant  Value=9
  Product1 : Product  Inputs=3
  Product2 : Product  Inputs=3
  Product6 : Product
  reaction enth (kj/molH2) : Constant  Value=-64
  Qreact : Outport
  F_molH2 : Outport  Port=2
  wires:
  9H2/1 -> Product2/2, Product1/3
  VolR/1 -> Product2/1, Product1/1
  rA (mol/m3 min)/1 -> Product1/2
  reaction enth (kj/molH2)/1 -> Product6/2
  Product1/1 -> F_molH2/1, Product6/1  "rA rate of H2 react (mol of H2/min)"
  Product6/1 -> Qreact/1  "dREact"
  Cb/1 -> Product2/3  "mol/m3min"

== system Research_project_CSTR_cascade/CSTR6/Hydrogen balance ==
  T-Tref : Inport
  FmolH2 : Inport  Port=2
  CpH2 : Inport  Port=3
  Constant1 : Constant  Value=Xout
  FoutH2CpdT2 : Product  Inputs=4
  N_H2*Cp : Product
  Scope1 : Scope
  QH2out : Outport
  N_h2*Cp : Outport  Port=2
  wires:
  FoutH2CpdT2/1 -> Scope1/1, QH2out/1  "QH2"
  T-Tref/1 -> FoutH2CpdT2/1
  CpH2/1 -> N_H2*Cp/2, FoutH2CpdT2/2
  FmolH2/1 -> N_H2*Cp/1, FoutH2CpdT2/3
  N_H2*Cp/1 -> N_h2*Cp/1  "QH2"
  Constant1/1 -> FoutH2CpdT2/4

== system Research_project_CSTR_cascade/CSTR6/Jacket ==
  In1 : Inport
  Area Heat (m2) : Constant  Value=A
  Q : Product  Inputs=3
  U (Kj/min m2 K) : Constant  Value=U
  Out1 : Outport
  wires:
  Area Heat (m2)/1 -> Q/3  "A jacket (m2)"
  U (Kj/min m2 K)/1 -> Q/1
  In1/1 -> Q/2  "T-Tjacket"
  Q/1 -> Out1/1  "Qjacket"

== system Research_project_CSTR_cascade/CSTR6/Kinetics ==
  T_Reactor (K) : Inport
  "A constant " : Math
  Constant : Constant  Value=37.634
  Ea (kj/mol) : Constant  Value=-204.68
  Effectiveness factor : Constant
  Math Function : Math
  Product3 : Product
  Product4 : Product  Inputs=3
  Product5 : Product  Inputs=*/
  R (kj/mol K) : Constant  Value=0.00831
  Rateconstant : Outport
  wires:
  T_Reactor (K)/1 -> Product3/1
  "A constant "/1 -> Product4/1
  Product3/1 -> Product5/2
  Constant/1 -> "A constant "/1
  Ea (kj/mol)/1 -> Product5/1
  Math Function/1 -> Product4/2
  R (kj/mol K)/1 -> Product3/2
  Product5/1 -> Math Function/1
  Product4/1 -> Rateconstant/1  "(min-1)"
  Effectiveness factor/1 -> Product4/3

== system Research_project_CSTR_cascade/CSTR6/Mass balance A ==
  v0/V : Inport
  rA : Inport  Port=2
  CA0 : Inport  Port=3
  Product1 : Product
  Scope : Scope
  Sum1 : Sum  Inputs=|+-
  Sum2 : Sum  Inputs=|+-
  dCa/dt : Integrator  InitialConditionSource=external  InitialCondition=3100
  Caout : Outport
  wires:
  rA/1 -> Sum2/2  "rA (mol/min m3)"
  Sum2/1 -> dCa/dt/1
  CA0/1 -> dCa/dt/2, Sum1/1
  Product1/1 -> Sum2/1
  dCa/dt/1 -> Scope/1, Caout/1, Sum1/2  "Ca (mol/m3 min)"
  Sum1/1 -> Product1/2  "Ca0-Ca"
  v0/V/1 -> Product1/1

== system Research_project_CSTR_cascade/CSTR6/Mass balance B ==
  v0/V : Inport
  rA : Inport  Port=2
  Cb0 : Inport  Port=3
  Product1 : Product
  Scope : Scope
  Sum1 : Sum  Inputs=|+-
  Sum2 : Sum  Inputs=|++
  dCb/dt : Integrator  InitialConditionSource=external  InitialCondition=3100
  Cbout : Outport
  wires:
  rA/1 -> Sum2/2  "rA (mol/min m3)"
  Sum2/1 -> dCb/dt/1
  Cb0/1 -> dCb/dt/2, Sum1/1
  Product1/1 -> Sum2/1
  dCb/dt/1 -> Scope/1, Cbout/1, Sum1/2  "Cb (mol/m3 min)"
  Sum1/1 -> Product1/2  "Cb0-Cb"
  v0/V/1 -> Product1/1

== system Research_project_CSTR_cascade/CSTR7/Energy dehydro ==
  VolR : Inport
  rA (mol/m3 min) : Inport  Port=2
  Cb : Inport  Port=3
  9H2 : Constant  Value=9
  Product1 : Product  Inputs=3
  Product2 : Product  Inputs=3
  Product6 : Product
  reaction enth (kj/molH2) : Constant  Value=-64
  Qreact : Outport
  F_molH2 : Outport  Port=2
  wires:
  9H2/1 -> Product2/2, Product1/3
  VolR/1 -> Product2/1, Product1/1
  rA (mol/m3 min)/1 -> Product1/2
  reaction enth (kj/molH2)/1 -> Product6/2
  Product1/1 -> F_molH2/1, Product6/1  "rA rate of H2 react (mol of H2/min)"
  Product6/1 -> Qreact/1  "dREact"
  Cb/1 -> Product2/3  "mol/m3min"

== system Research_project_CSTR_cascade/CSTR7/Hydrogen balance ==
  T-Tref : Inport
  FmolH2 : Inport  Port=2
  CpH2 : Inport  Port=3
  Constant1 : Constant  Value=Xout
  FoutH2CpdT2 : Product  Inputs=4
  N_H2*Cp : Product
  Scope1 : Scope
  QH2out : Outport
  N_h2*Cp : Outport  Port=2
  wires:
  FoutH2CpdT2/1 -> Scope1/1, QH2out/1  "QH2"
  T-Tref/1 -> FoutH2CpdT2/1
  CpH2/1 -> N_H2*Cp/2, FoutH2CpdT2/2
  FmolH2/1 -> N_H2*Cp/1, FoutH2CpdT2/3
  N_H2*Cp/1 -> N_h2*Cp/1  "QH2"
  Constant1/1 -> FoutH2CpdT2/4

== system Research_project_CSTR_cascade/CSTR7/Jacket ==
  In1 : Inport
  Area Heat (m2) : Constant  Value=A
  Q : Product  Inputs=3
  U (Kj/min m2 K) : Constant  Value=U
  Out1 : Outport
  wires:
  Area Heat (m2)/1 -> Q/3  "A jacket (m2)"
  U (Kj/min m2 K)/1 -> Q/1
  In1/1 -> Q/2  "T-Tjacket"
  Q/1 -> Out1/1  "Qjacket"

== system Research_project_CSTR_cascade/CSTR7/Kinetics ==
  T_Reactor (K) : Inport
  "A constant " : Math
  Constant : Constant  Value=37.634
  Ea (kj/mol) : Constant  Value=-204.68
  Effectiveness factor : Constant
  Math Function : Math
  Product3 : Product
  Product4 : Product  Inputs=3
  Product5 : Product  Inputs=*/
  R (kj/mol K) : Constant  Value=0.00831
  Rateconstant : Outport
  wires:
  T_Reactor (K)/1 -> Product3/1
  "A constant "/1 -> Product4/1
  Product3/1 -> Product5/2
  Constant/1 -> "A constant "/1
  Ea (kj/mol)/1 -> Product5/1
  Math Function/1 -> Product4/2
  R (kj/mol K)/1 -> Product3/2
  Product5/1 -> Math Function/1
  Product4/1 -> Rateconstant/1  "(min-1)"
  Effectiveness factor/1 -> Product4/3

== system Research_project_CSTR_cascade/CSTR7/Mass balance A ==
  v0/V : Inport
  rA : Inport  Port=2
  CA0 : Inport  Port=3
  Product1 : Product
  Scope : Scope
  Sum1 : Sum  Inputs=|+-
  Sum2 : Sum  Inputs=|+-
  dCa/dt : Integrator  InitialConditionSource=external  InitialCondition=3100
  Caout : Outport
  wires:
  rA/1 -> Sum2/2  "rA (mol/min m3)"
  Sum2/1 -> dCa/dt/1
  CA0/1 -> dCa/dt/2, Sum1/1
  Product1/1 -> Sum2/1
  dCa/dt/1 -> Scope/1, Caout/1, Sum1/2  "Ca (mol/m3 min)"
  Sum1/1 -> Product1/2  "Ca0-Ca"
  v0/V/1 -> Product1/1

== system Research_project_CSTR_cascade/CSTR7/Mass balance B ==
  v0/V : Inport
  rA : Inport  Port=2
  Cb0 : Inport  Port=3
  Product1 : Product
  Scope : Scope
  Sum1 : Sum  Inputs=|+-
  Sum2 : Sum  Inputs=|++
  dCb/dt : Integrator  InitialConditionSource=external  InitialCondition=3100
  Cbout : Outport
  wires:
  rA/1 -> Sum2/2  "rA (mol/min m3)"
  Sum2/1 -> dCb/dt/1
  Cb0/1 -> dCb/dt/2, Sum1/1
  Product1/1 -> Sum2/1
  dCb/dt/1 -> Scope/1, Cbout/1, Sum1/2  "Cb (mol/m3 min)"
  Sum1/1 -> Product1/2  "Cb0-Cb"
  v0/V/1 -> Product1/1

== system Research_project_CSTR_cascade/CSTR8/Energy dehydro ==
  VolR : Inport
  rA (mol/m3 min) : Inport  Port=2
  Cb : Inport  Port=3
  9H2 : Constant  Value=9
  Product1 : Product  Inputs=3
  Product2 : Product  Inputs=3
  Product6 : Product
  reaction enth (kj/molH2) : Constant  Value=-64
  Qreact : Outport
  F_molH2 : Outport  Port=2
  wires:
  9H2/1 -> Product2/2, Product1/3
  VolR/1 -> Product2/1, Product1/1
  rA (mol/m3 min)/1 -> Product1/2
  reaction enth (kj/molH2)/1 -> Product6/2
  Product1/1 -> F_molH2/1, Product6/1  "rA rate of H2 react (mol of H2/min)"
  Product6/1 -> Qreact/1  "dREact"
  Cb/1 -> Product2/3  "mol/m3min"

== system Research_project_CSTR_cascade/CSTR8/Hydrogen balance ==
  T-Tref : Inport
  FmolH2 : Inport  Port=2
  CpH2 : Inport  Port=3
  Constant1 : Constant  Value=Xout
  FoutH2CpdT2 : Product  Inputs=4
  N_H2*Cp : Product
  Scope1 : Scope
  QH2out : Outport
  N_h2*Cp : Outport  Port=2
  wires:
  FoutH2CpdT2/1 -> Scope1/1, QH2out/1  "QH2"
  T-Tref/1 -> FoutH2CpdT2/1
  CpH2/1 -> N_H2*Cp/2, FoutH2CpdT2/2
  FmolH2/1 -> N_H2*Cp/1, FoutH2CpdT2/3
  N_H2*Cp/1 -> N_h2*Cp/1  "QH2"
  Constant1/1 -> FoutH2CpdT2/4

== system Research_project_CSTR_cascade/CSTR8/Jacket ==
  In1 : Inport
  Area Heat (m2) : Constant  Value=A
  Q : Product  Inputs=3
  U (Kj/min m2 K) : Constant  Value=U
  Out1 : Outport
  wires:
  Area Heat (m2)/1 -> Q/3  "A jacket (m2)"
  U (Kj/min m2 K)/1 -> Q/1
  In1/1 -> Q/2  "T-Tjacket"
  Q/1 -> Out1/1  "Qjacket"

== system Research_project_CSTR_cascade/CSTR8/Kinetics ==
  T_Reactor (K) : Inport
  "A constant " : Math
  Constant : Constant  Value=37.634
  Ea (kj/mol) : Constant  Value=-204.68
  Effectiveness factor : Constant
  Math Function : Math
  Product3 : Product
  Product4 : Product  Inputs=3
  Product5 : Product  Inputs=*/
  R (kj/mol K) : Constant  Value=0.00831
  Rateconstant : Outport
  wires:
  T_Reactor (K)/1 -> Product3/1
  "A constant "/1 -> Product4/1
  Product3/1 -> Product5/2
  Constant/1 -> "A constant "/1
  Ea (kj/mol)/1 -> Product5/1
  Math Function/1 -> Product4/2
  R (kj/mol K)/1 -> Product3/2
  Product5/1 -> Math Function/1
  Product4/1 -> Rateconstant/1  "(min-1)"
  Effectiveness factor/1 -> Product4/3

== system Research_project_CSTR_cascade/CSTR8/Mass balance A ==
  v0/V : Inport
  rA : Inport  Port=2
  CA0 : Inport  Port=3
  Product1 : Product
  Scope : Scope
  Sum1 : Sum  Inputs=|+-
  Sum2 : Sum  Inputs=|+-
  dCa/dt : Integrator  InitialConditionSource=external  InitialCondition=3100
  Caout : Outport
  wires:
  rA/1 -> Sum2/2  "rA (mol/min m3)"
  Sum2/1 -> dCa/dt/1
  CA0/1 -> dCa/dt/2, Sum1/1
  Product1/1 -> Sum2/1
  dCa/dt/1 -> Scope/1, Caout/1, Sum1/2  "Ca (mol/m3 min)"
  Sum1/1 -> Product1/2  "Ca0-Ca"
  v0/V/1 -> Product1/1

== system Research_project_CSTR_cascade/CSTR8/Mass balance B ==
  v0/V : Inport
  rA : Inport  Port=2
  Cb0 : Inport  Port=3
  Product1 : Product
  Scope : Scope
  Sum1 : Sum  Inputs=|+-
  Sum2 : Sum  Inputs=|++
  dCb/dt : Integrator  InitialConditionSource=external  InitialCondition=3100
  Cbout : Outport
  wires:
  rA/1 -> Sum2/2  "rA (mol/min m3)"
  Sum2/1 -> dCb/dt/1
  Cb0/1 -> dCb/dt/2, Sum1/1
  Product1/1 -> Sum2/1
  dCb/dt/1 -> Scope/1, Cbout/1, Sum1/2  "Cb (mol/m3 min)"
  Sum1/1 -> Product1/2  "Cb0-Cb"
  v0/V/1 -> Product1/1

== system Research_project_CSTR_cascade/CSTR9/Energy dehydro ==
  VolR : Inport
  rA (mol/m3 min) : Inport  Port=2
  Cb : Inport  Port=3
  9H2 : Constant  Value=9
  Product1 : Product  Inputs=3
  Product2 : Product  Inputs=3
  Product6 : Product
  reaction enth (kj/molH2) : Constant  Value=-64
  Qreact : Outport
  F_molH2 : Outport  Port=2
  wires:
  9H2/1 -> Product2/2, Product1/3
  VolR/1 -> Product2/1, Product1/1
  rA (mol/m3 min)/1 -> Product1/2
  reaction enth (kj/molH2)/1 -> Product6/2
  Product1/1 -> F_molH2/1, Product6/1  "rA rate of H2 react (mol of H2/min)"
  Product6/1 -> Qreact/1  "dREact"
  Cb/1 -> Product2/3  "mol/m3min"

== system Research_project_CSTR_cascade/CSTR9/Hydrogen balance ==
  T-Tref : Inport
  FmolH2 : Inport  Port=2
  CpH2 : Inport  Port=3
  Constant1 : Constant  Value=Xout
  FoutH2CpdT2 : Product  Inputs=4
  N_H2*Cp : Product
  Scope1 : Scope
  QH2out : Outport
  N_h2*Cp : Outport  Port=2
  wires:
  FoutH2CpdT2/1 -> Scope1/1, QH2out/1  "QH2"
  T-Tref/1 -> FoutH2CpdT2/1
  CpH2/1 -> N_H2*Cp/2, FoutH2CpdT2/2
  FmolH2/1 -> N_H2*Cp/1, FoutH2CpdT2/3
  N_H2*Cp/1 -> N_h2*Cp/1  "QH2"
  Constant1/1 -> FoutH2CpdT2/4

== system Research_project_CSTR_cascade/CSTR9/Jacket ==
  In1 : Inport
  Area Heat (m2) : Constant  Value=A
  Q : Product  Inputs=3
  U (Kj/min m2 K) : Constant  Value=U
  Out1 : Outport
  wires:
  Area Heat (m2)/1 -> Q/3  "A jacket (m2)"
  U (Kj/min m2 K)/1 -> Q/1
  In1/1 -> Q/2  "T-Tjacket"
  Q/1 -> Out1/1  "Qjacket"

== system Research_project_CSTR_cascade/CSTR9/Kinetics ==
  T_Reactor (K) : Inport
  "A constant " : Math
  Constant : Constant  Value=37.634
  Ea (kj/mol) : Constant  Value=-204.68
  Effectiveness factor : Constant
  Math Function : Math
  Product3 : Product
  Product4 : Product  Inputs=3
  Product5 : Product  Inputs=*/
  R (kj/mol K) : Constant  Value=0.00831
  Rateconstant : Outport
  wires:
  T_Reactor (K)/1 -> Product3/1
  "A constant "/1 -> Product4/1
  Product3/1 -> Product5/2
  Constant/1 -> "A constant "/1
  Ea (kj/mol)/1 -> Product5/1
  Math Function/1 -> Product4/2
  R (kj/mol K)/1 -> Product3/2
  Product5/1 -> Math Function/1
  Product4/1 -> Rateconstant/1  "(min-1)"
  Effectiveness factor/1 -> Product4/3

== system Research_project_CSTR_cascade/CSTR9/Mass balance A ==
  v0/V : Inport
  rA : Inport  Port=2
  CA0 : Inport  Port=3
  Product1 : Product
  Scope : Scope
  Sum1 : Sum  Inputs=|+-
  Sum2 : Sum  Inputs=|+-
  dCa/dt : Integrator  InitialConditionSource=external  InitialCondition=3100
  Caout : Outport
  wires:
  rA/1 -> Sum2/2  "rA (mol/min m3)"
  Sum2/1 -> dCa/dt/1
  CA0/1 -> dCa/dt/2, Sum1/1
  Product1/1 -> Sum2/1
  dCa/dt/1 -> Scope/1, Caout/1, Sum1/2  "Ca (mol/m3 min)"
  Sum1/1 -> Product1/2  "Ca0-Ca"
  v0/V/1 -> Product1/1

== system Research_project_CSTR_cascade/CSTR9/Mass balance B ==
  v0/V : Inport
  rA : Inport  Port=2
  Cb0 : Inport  Port=3
  Product1 : Product
  Scope : Scope
  Sum1 : Sum  Inputs=|+-
  Sum2 : Sum  Inputs=|++
  dCb/dt : Integrator  InitialConditionSource=external  InitialCondition=3100
  Cbout : Outport
  wires:
  rA/1 -> Sum2/2  "rA (mol/min m3)"
  Sum2/1 -> dCb/dt/1
  Cb0/1 -> dCb/dt/2, Sum1/1
  Product1/1 -> Sum2/1
  dCb/dt/1 -> Scope/1, Cbout/1, Sum1/2  "Cb (mol/m3 min)"
  Sum1/1 -> Product1/2  "Cb0-Cb"
  v0/V/1 -> Product1/1
